simulink model "B5_simulation_paparazzi"  (R2021b)
settings: Solver=VariableStepAuto  StartTime=0.0  StopTime=5.5  FixedStep=0.002  RelTol=1e-3
values from neighbouring files (symbols this model uses):
  coef_sim_1 = tf_des_d.Denominator{1}(2)    [A11_setup_script_pprz.m]    (also in A1_setup_script.m; A6_slow_actuator.m)
  coef_sim_2 = tf_des_d.Numerator{1}(2)    [A11_setup_script_pprz.m]    (also in A1_setup_script.m; A6_slow_actuator.m)
  coeff = 1    [A11_setup_script_pprz.m]    (also in A12_sim_multi_run.m = coeff_list(i))
  doublet_mag = - 0.15    (= -0.15)    [A11_setup_script_pprz.m]    (also in A1_setup_script.m)
  doublet_time = 6    [A11_setup_script_pprz.m]    (also in A1_setup_script.m)
  f_8 = 1    [A11_setup_script_pprz.m]    (also in A1_setup_script.m)
  FILT_CUTOFF = 2*pi*5    (= 31.4159265359)    [A11_setup_script_pprz.m]    (also in A1_setup_script.m)
  FILTER = 1    [A11_setup_script_pprz.m]    (also in A1_setup_script.m)
  G1 = inv(I)*G1_r    [A10_simple_plant.m]    (also in A11_setup_script_pprz.m = G1/scale; A1_setup_script.m = [G1;G1_T])
  G2 = G2/scale    [A11_setup_script_pprz.m]    (also in A1_setup_script.m = (1/sampling_time)*inv(I)*(G2_r))
  h_plate = 0.3    [A11_setup_script_pprz.m]    (also in A1_setup_script.m = 0.16)
  I = eye(3,3)    [A10_simple_plant.m]    (also in A11_setup_script_pprz.m; A1_setup_script.m; A2_B_matrix_generation_symbolic.m = [Ixx 0 0; A3_B_matrix_generation_symbolic_cascaded.m = [Ixx 0 0)
  Iyy = 0.0008    [A11_setup_script_pprz.m]    (also in A1_setup_script.m = 0.0015)
  K = 7    [A11_setup_script_pprz.m]    (also in A1_setup_script.m = 10)
  K_act = 50    [A10_simple_plant.m]    (also in A11_setup_script_pprz.m = 20; A1_setup_script.m = 20)
  K_d = 15    [A11_setup_script_pprz.m]    (also in A1_setup_script.m = 25)
  K_dd = K_act    (= 20)    [A11_setup_script_pprz.m]    (also in A1_setup_script.m)
  K_ec = 50    [A11_setup_script_pprz.m]    (also in A1_setup_script.m = 251)
  K_ec_d = 13    [A11_setup_script_pprz.m]    (also in A1_setup_script.m = 25)
  K_ec_d_u = 1.5    [A11_setup_script_pprz.m]    (also in A1_setup_script.m = 5)
  K_ec_d_v = 1.5    [A11_setup_script_pprz.m]    (also in A1_setup_script.m = 5)
  K_ec_dd = 9    [A11_setup_script_pprz.m]    (also in A1_setup_script.m = 45)
  K_ec_i = 0    [A11_setup_script_pprz.m]    (also in A1_setup_script.m = 380)
  K_ec_u = 1.5    [A11_setup_script_pprz.m]    (also in A1_setup_script.m = 5)
  K_ec_v = 1.5    [A11_setup_script_pprz.m]    (also in A1_setup_script.m = 5)
  K_t = 0.0005    [A10_simple_plant.m]    (also in A11_setup_script_pprz.m = 6.557e-08; A1_setup_script.m = 6.557e-08)
  K_u = 1.0    (= 1)    [A11_setup_script_pprz.m]    (also in A1_setup_script.m = 1.5)
  K_u_d = 2.5    [A11_setup_script_pprz.m]    (also in A1_setup_script.m = 7)
  K_v = 1.0    (= 1)    [A11_setup_script_pprz.m]    (also in A1_setup_script.m = 1.5)
  K_v_d = 2.5    [A11_setup_script_pprz.m]    (also in A1_setup_script.m = 7)
  K_w = 1.0    (= 1)    [A11_setup_script_pprz.m]    (also in A1_setup_script.m = 4.5)
  K_w_d = 2.5    [A11_setup_script_pprz.m]    (also in A1_setup_script.m = 7)
  l_plate = 0.1    [A11_setup_script_pprz.m]    (also in A1_setup_script.m = 0.11)
  m = 0.4    [A10_simple_plant.m]    (also in A11_setup_script_pprz.m; A1_setup_script.m)
  NOISE = 0    [A11_setup_script_pprz.m]    (also in A1_setup_script.m)
  NOISE_ACC = 0.00005    (= 5e-05)    [A11_setup_script_pprz.m]    (also in A1_setup_script.m)
  NOISE_GYRO = 0.00005    (= 5e-05)    [A11_setup_script_pprz.m]    (also in A1_setup_script.m)
  NOISE_RPM = 200    [A11_setup_script_pprz.m]    (also in A1_setup_script.m)
  omega_des = 20.00    (= 20)    [A11_setup_script_pprz.m]    (also in A1_setup_script.m; A6_slow_actuator.m = 49)
  sampling_time = 1/frequency    (= 0.002)    [A11_setup_script_pprz.m]    (also in A12_sim_multi_run.m; A1_setup_script.m; A6_slow_actuator.m)
  scale_8 = 1.6    [A11_setup_script_pprz.m]    (also in A1_setup_script.m)
  start_8 = 2    [A11_setup_script_pprz.m]    (also in A1_setup_script.m)
  start_time = 2    [A11_setup_script_pprz.m]    (also in A1_setup_script.m = 1)
  t_8 = 10    [A11_setup_script_pprz.m]    (also in A1_setup_script.m)
  w_plate = 0.3    [A11_setup_script_pprz.m]    (also in A1_setup_script.m = 0.36)
undefined symbols (not defined in the file or in its folder): DiscIntNeverNeededParam
libraries: simulink x11, cstblocks x9, dspinverses x8, dspmathops x4, dspstat3 x4, aerolibutil x3, sharedutil x2, aerolibanim x1
(part 3 of 5)

== system B5_simulation_paparazzi/Model Block Complementary Filters/Simple INDI/INTERNAL REFERENCE MODEL ATTITUDE ==
  phi_cmd : Inport
  theta_cmd : Inport  Port=2
  psi_cmd : Inport  Port=3
  Discrete-Time Integrator{,1..8} (9 alike) : DiscreteIntegrator  SampleTime=sampling_time  ICPrevOutput=DiscIntNeverNeededParam  ICPrevScaledInput=DiscIntNeverNeededParam
  Gain1 : Gain  Gain=K
  Gain2 : Gain  Gain=K_dd
  Gain3 : Gain  Gain=K
  Gain4 : Gain  Gain=K_d
  Gain5 : Gain  Gain=K_d
  Gain6 : Gain  Gain=K_d
  Gain7 : Gain  Gain=K
  Gain8 : Gain  Gain=K_dd
  Gain9 : Gain  Gain=K_dd
  MATLAB Function1 : MATLAB Function  TreatAsAtomicUnit=on
  Mux : Mux  Inputs=6
  Scope : Scope  NumInputPorts=2
  Sum{1..4,11,16,20..22} (9 alike) : Sum  Inputs=|+-
  To Workspace : ToWorkspace  VariableName=simout  SaveFormat=Timeseries  SampleTime=-1
  body rates to euler rates : Subsystem
  euler rates to body rates : Subsystem
  pd_ref : Outport
  qd_ref : Outport  Port=2
  rd_ref : Outport  Port=3
  p_ref : Outport  Port=4
  q_ref : Outport  Port=5
  r_ref : Outport  Port=6
  phi_ref : Outport  Port=7
  theta_ref : Outport  Port=8
  psi_ref : Outport  Port=9
  tag scope: p_ref=global, phi_ref=global, psi_ref=global, q_ref=global, r_ref=global, theta_ref=global
  wires:
  Discrete-Time Integrator5/1 -> [r_ref], r_ref/1, body rates to euler rates/3(r), Sum22/2  "r_ref"
  [qd_f] -> Mux/4
  MATLAB Function1/1(psie_w) -> Gain3/1  "wrapped_Err"
  Sum22/1 -> Gain6/1
  euler rates to body rates/3(r) -> Sum22/1
  Sum4/1 -> Gain9/1
  Gain1/1 -> euler rates to body rates/2(theta_dot)
  Discrete-Time Integrator7/1 -> Sum3/2, Discrete-Time Integrator4/1, Mux/1, qd_ref/1  "qd_ref"
  Mux/1 -> To Workspace/1
  psi_cmd/1 -> Sum1/1  "psi_cmd"
  Gain9/1 -> Discrete-Time Integrator8/1  "rdd_ref"
  theta_cmd/1 -> Sum11/1  "theta_cmd"
  Gain4/1 -> Sum2/1
  Sum1/1 -> MATLAB Function1/1(pis_e)  "err"
  Discrete-Time Integrator/1 -> [psi_ref], psi_ref/1, Sum1/2  "psi_ref"
  Sum2/1 -> Gain2/1
  Gain3/1 -> euler rates to body rates/3(psi_dot)
  body rates to euler rates/2(theta_dot) -> Scope/2, Discrete-Time Integrator1/1
  Discrete-Time Integrator2/1 -> [phi_ref], phi_ref/1, Sum20/2  "phi_ref"
  Gain6/1 -> Sum4/1
  Sum20/1 -> Gain7/1
  Gain8/1 -> Discrete-Time Integrator7/1  "qdd_ref"
  euler rates to body rates/1(p) -> Sum21/1
  Sum11/1 -> Gain1/1
  Gain2/1 -> Discrete-Time Integrator6/1  "pdd_ref"
  Sum21/1 -> Gain4/1
  Discrete-Time Integrator1/1 -> [theta_ref], Mux/3, theta_ref/1, Sum11/2  "theta_ref"
  Sum3/1 -> Gain8/1
  Gain5/1 -> Sum3/1
  Discrete-Time Integrator6/1 -> Sum2/2, Discrete-Time Integrator3/1, pd_ref/1  "pd_ref"
  euler rates to body rates/2(q) -> Sum16/1
  [theta] -> Mux/6
  Discrete-Time Integrator8/1 -> Sum4/2, Discrete-Time Integrator5/1, rd_ref/1  "rd_ref"
  body rates to euler rates/3(psi_dot) -> Discrete-Time Integrator/1
  phi_cmd/1 -> Sum20/1  "phi_cmd"
  body rates to euler rates/1(phi_dot) -> Discrete-Time Integrator2/1
  [q] -> Mux/5
  Gain7/1 -> euler rates to body rates/1(phi_dot)
  Discrete-Time Integrator3/1 -> [p_ref], p_ref/1, body rates to euler rates/1(p), Sum21/2  "p_ref"
  Discrete-Time Integrator4/1 -> Scope/1, body rates to euler rates/2(q), [q_ref], Mux/2, q_ref/1, Sum16/2  "q_ref"
  Sum16/1 -> Gain5/1

== system B5_simulation_paparazzi/Model Block Complementary Filters/Simple INDI/INTERNAL REFERENCE MODEL VELOCITY ==
  Vx_cmd : Inport
  Vy_cmd : Inport  Port=2
  Vz_cmd : Inport  Port=3
  Discrete-Time Integrator{,1..5} (6 alike) : DiscreteIntegrator  SampleTime=-1  ICPrevOutput=DiscIntNeverNeededParam  ICPrevScaledInput=DiscIntNeverNeededParam
  Gain1 : Gain  Gain=K_w_d
  Gain2 : Gain  Gain=K_v_d
  Gain3 : Gain  Gain=K_w
  Gain4 : Gain  Gain=K_v
  Gain5 : Gain  Gain=K_u
  Gain9 : Gain  Gain=K_u_d
  Sum{1..4,11,20} (6 alike) : Sum  Inputs=|+-
  Ax_ref : Outport
  Ay_ref : Outport  Port=2
  Az_ref : Outport  Port=3
  Vx_ref : Outport  Port=4
  Vy_ref : Outport  Port=5
  Vz_ref : Outport  Port=6
  X_ref : Outport  Port=7
  Y_ref : Outport  Port=8
  Z_ref : Outport  Port=9
  tag scope: Ax_ref=global, Ay_ref=global, Az_ref=global, Vx_ref=global, Vy_ref=global, Vz_ref=global
  wires:
  Discrete-Time Integrator1/1 -> Sum3/2, Discrete-Time Integrator4/1, [Vy_ref], Vz_ref/1
  Gain1/1 -> Discrete-Time Integrator1/1, [Az_ref], Az_ref/1
  Gain9/1 -> Discrete-Time Integrator/1, [Ax_ref], Ax_ref/1
  Vy_cmd/1 -> Sum1/1
  Discrete-Time Integrator/1 -> Sum4/2, Discrete-Time Integrator3/1, [Vx_ref], Vx_ref/1
  Vx_cmd/1 -> Sum20/1
  Vz_cmd/1 -> Sum11/1
  Discrete-Time Integrator2/1 -> Sum2/2, Discrete-Time Integrator5/1, [Vz_ref], Vy_ref/1
  Gain2/1 -> Discrete-Time Integrator2/1, [Ay_ref], Ay_ref/1
  Sum20/1 -> Gain5/1
  Sum11/1 -> Gain3/1
  Sum1/1 -> Gain4/1
  Gain4/1 -> Sum2/1
  Gain3/1 -> Sum3/1
  Gain5/1 -> Sum4/1
  Sum3/1 -> Gain1/1
  Sum2/1 -> Gain2/1
  Sum4/1 -> Gain9/1
  Discrete-Time Integrator3/1 -> X_ref/1, Sum20/2
  Discrete-Time Integrator4/1 -> Sum11/2, Z_ref/1
  Discrete-Time Integrator5/1 -> Sum1/2, Y_ref/1

== system B5_simulation_paparazzi/Model Block Normal Filters/Continuous Actuator Dynamics/Butterworth Lowpass 2nd Order1 ==
  In : Inport
  Constant : Constant  Value=FILTER  SampleTime=sampling_time
  Merge : Merge
  Switch Case : SwitchCase
  Switch Case Action Subsystem : Subsystem  TreatAsAtomicUnit=on
  Switch Case Action Subsystem1 : Subsystem  TreatAsAtomicUnit=on
  Out : Outport
  wires:
  Merge/1 -> Out/1
  Switch Case Action Subsystem/1(Out1) -> Merge/1
  Constant/1 -> Switch Case/1
  Switch Case Action Subsystem1/1(Out1) -> Merge/2
  Switch Case/2 -> Switch Case Action Subsystem1/Action
  In/1 -> Switch Case Action Subsystem/1(In1), Switch Case Action Subsystem1/1(In1)
  Switch Case/1 -> Switch Case Action Subsystem/Action

== system B5_simulation_paparazzi/Model Block Normal Filters/Continuous Actuator Dynamics/Noise RPM ==
  Constant : Constant  Value=NOISE  SampleTime=sampling_time
  Merge : Merge
  Switch Case : SwitchCase
  Switch Case Action Subsystem : Subsystem  TreatAsAtomicUnit=on
  Switch Case Action Subsystem1 : Subsystem  TreatAsAtomicUnit=on
  Out : Outport
  wires:
  Switch Case/2 -> Switch Case Action Subsystem1/Action
  Merge/1 -> Out/1
  Switch Case/1 -> Switch Case Action Subsystem/Action
  Constant/1 -> Switch Case/1
  Switch Case Action Subsystem1/1(Out1) -> Merge/2
  Switch Case Action Subsystem/1(Out1) -> Merge/1

== system B5_simulation_paparazzi/Model Block Normal Filters/Extended INDI/8-shape trajectory ==
  Abs : Abs
  Abs1 : Abs
  Clock : Clock
      settings: Decimation=100
  Constant : Constant  Value=f_8
  Constant1 : Constant  Value=scale_8
  Constant2 : Constant  Value=t_8
  Constant3 : Constant  Value=sampling_time
  Constant4 : Constant  Value=0
  Constant5 : Constant  Value=start_8
  Constant6 : Constant  Value=t_8
  Constant7 : Constant  Value=start_8
  Integrator : Integrator
  MATLAB Function : MATLAB Function  TreatAsAtomicUnit=on
  Scope : Scope
  Scope1 : Scope
  Sum : Sum  Inputs=|+-
  Sum3 : Sum  Inputs=|+-
  Sum7 : Sum  Inputs=|+-
  Sum9 : Sum  Inputs=|++
  Switch : Switch  Criteria=u2 > Threshold  Threshold=t_8
  Switch1 : Switch  Criteria=u2 > Threshold  Threshold=start_8
  Zero-Order Hold : ZeroOrderHold  SampleTime=sampling_time
  x_traj : Outport
  y_traj : Outport  Port=2
  psi_traj : Outport  Port=3
  wires:
  Constant2/1 -> Switch/1
  Switch/1 -> Scope/1, MATLAB Function/1(t)  "t"
  Constant/1 -> MATLAB Function/2(f)
  MATLAB Function/2(y) -> y_traj/1, Sum7/2  "y_traj"
  Zero-Order Hold/1 -> Switch/2, Switch/3
  Constant1/1 -> MATLAB Function/3(scale)
  Constant3/1 -> MATLAB Function/4(sampling_time)
  MATLAB Function/1(x) -> x_traj/1, Sum3/2  "x_traj"
  MATLAB Function/3(psi) -> psi_traj/1  "psi_traj"
  Clock/1 -> Sum/1, Switch1/2
  Constant4/1 -> Switch1/3
  Switch1/1 -> Zero-Order Hold/1
  Constant5/1 -> Sum/2
  Sum/1 -> Switch1/1
  Constant6/1 -> MATLAB Function/5(total_time)
  Sum7/1 -> Abs1/1
  Abs/1 -> Sum9/1
  Abs1/1 -> Sum9/2
  [y] -> Sum7/1
  Sum9/1 -> Integrator/1
  Integrator/1 -> Scope1/1  "pos_err"
  [x] -> Sum3/1
  Sum3/1 -> Abs/1
  Constant7/1 -> MATLAB Function/6(start_time)

== system B5_simulation_paparazzi/Model Block Normal Filters/Extended INDI/Doublet Block ==
  Scope : Scope
  Step : Step  Time=start_time  After=doublet_mag  SampleTime=sampling_time
  Step1 : Step  Time=start_time + doublet_time/2  After=-doublet_mag*2  SampleTime=sampling_time
  Step2 : Step  Time=start_time + doublet_time  After=doublet_mag  SampleTime=sampling_time
  Sum : Sum  Inputs=|++
  Sum1 : Sum  Inputs=|++
  theta_cmd : Outport
  wires:
  Step/1 -> Sum/1
  Step1/1 -> Sum/2
  Sum/1 -> Sum1/1
  Sum1/1 -> theta_cmd/1, Scope/1
  Step2/1 -> Sum1/2

== system B5_simulation_paparazzi/Model Block Normal Filters/Extended INDI/ERROR CONTROLLER ATTITUDE ==
  pd_ref : Inport
  qd_ref : Inport  Port=2
  rd_ref : Inport  Port=3
  p_ref : Inport  Port=4
  q_ref : Inport  Port=5
  r_ref : Inport  Port=6
  phi_ref : Inport  Port=7
  theta_ref : Inport  Port=8
  psi_ref : Inport  Port=9
  Abs : Abs
  Add : Sum  Inputs=++++
  Add1 : Sum  Inputs=++++
  Add2 : Sum  Inputs=++++
  Cumulative Sum : dspmathops/Cumulative Sum  dim=Channels (running sum)  InputProcessing=Columns as channels (frame based)  reset_popup=None  roundingMode=Floor  overflowMode=off  outputDataTypeStr=Inherit: Same as accumulator  outputMin=[]  outputMax=[]  outputLastDataTypeStr=Inherit: Same as accumulator
  Display : Display
  Display1 : Display
  Gain : Gain  Gain=K_ec_dd + K_act
  Gain1 : Gain  Gain=K_ec_d *(1 + K_act)
  Gain2 : Gain  Gain=K_ec*(1 + K_act)
  Gain3 : Gain  Gain=K_ec_dd + K_act
  Gain4 : Gain  Gain=K_ec_d *(1 + K_act)
  Gain5 : Gain  Gain=K_ec *(1 + K_act)
  Gain6 : Gain  Gain=K_ec_dd + K_act
  Gain7 : Gain  Gain=K_ec_d *(1 + K_act)
  Gain8 : Gain  Gain=K_ec *(1 + K_act)
  MATLAB Function1 : MATLAB Function  TreatAsAtomicUnit=on
  Mean : dspstat3/Mean  run=off  InputProcessing=Columns as channels (frame based)  reset_popup=None  directionMode=Each column  dimension=1  roiEnable=off  roiType=Rectangles  roiPortion=Entire ROI  roiOutput=Individual statistics for each ROI  roiFlag=off  roundingMode=Floor  overflowMode=off  outputDataTypeStr=Inherit: Same as accumulator  outputMin=[]  outputMax=[]  outputLastDataTypeStr=Inherit: Same as accumulator
  Scope : Scope  NumInputPorts=4
  Sum{,1..8} (9 alike) : Sum  Inputs=|+-
  pdd_ec : Outport
  qdd_ec : Outport  Port=2
  rdd_ec : Outport  Port=3
  wires:
  pd_ref/1 -> Sum/1
  p_ref/1 -> Sum1/1
  Add/1 -> pdd_ec/1
  [p] -> Sum1/2
  [phi] -> Sum2/2
  phi_ref/1 -> Sum2/1
  [pd_f] -> Sum/2
  Sum/1 -> Gain/1  "pd_err"
  Gain/1 -> Add/1
  Sum1/1 -> Gain1/1  "p_err"
  Sum2/1 -> Gain2/1  "phi_err"
  Gain1/1 -> Add/2
  Gain2/1 -> Add/3
  Sum4/1 -> Gain4/1  "q_err"
  [qd_f] -> Sum3/2
  Gain4/1 -> Add1/2
  Gain5/1 -> Add1/3
  theta_ref/1 -> Sum5/1
  [theta] -> Sum5/2
  [q] -> Sum4/2
  Gain3/1 -> Add1/1
  q_ref/1 -> Sum4/1
  Add1/1 -> qdd_ec/1
  qd_ref/1 -> Sum3/1
  Sum7/1 -> Gain7/1  "r_err"
  Sum8/1 -> MATLAB Function1/1(pis_e)
  Sum6/1 -> Gain6/1  "rd_err"
  [rd_f] -> Sum6/2
  Gain7/1 -> Scope/2, Add2/2  "2"
  Gain8/1 -> Scope/3, Add2/3  "3"
  psi_ref/1 -> Sum8/1
  [psi] -> Sum8/2
  [r] -> Sum7/2
  Gain6/1 -> Add2/1, Scope/1  "1"
  r_ref/1 -> Sum7/1
  Add2/1 -> rdd_ec/1
  rd_ref/1 -> Sum6/1
  Sum3/1 -> Gain3/1  "qd_err"
  Sum5/1 -> Abs/1, Gain5/1  "theta_err"
  MATLAB Function1/1(psie_w) -> Gain8/1  "psi_err"
  Abs/1 -> Mean/1, Cumulative Sum/1  "theta_err_abs"
  Cumulative Sum/1 -> Display/1
  Mean/1 -> Display1/1

== system B5_simulation_paparazzi/Model Block Normal Filters/Extended INDI/ERROR CONTROLLER VELOCITY ==
  Vx_ref : Inport
  Vy_ref : Inport  Port=2
  Vz_ref : Inport  Port=3
  X_ref : Inport  Port=4
  Y_ref : Inport  Port=5
  Z_ref : Inport  Port=6
  Gain : Gain  Gain=K_ec_u
  Gain1 : Gain  Gain=K_ec_d_u
  Gain2 : Gain  Gain=K_ec_v
  Gain3 : Gain  Gain=K_ec_d_v
  Gain4 : Gain  Gain=K_ec_v
  Gain5 : Gain  Gain=K_ec_d_v
  Sum{,3,5..8} (6 alike) : Sum  Inputs=|+-
  Sum1 : Sum  Inputs=|++
  Sum2 : Sum  Inputs=|++
  Sum4 : Sum  Inputs=|++
  Ax_ec : Outport
  Ay_ec : Outport  Port=2
  Az_ec : Outport  Port=3
  wires:
  [Vz] -> Sum6/2
  Sum1/1 -> Ax_ec/1
  Sum2/1 -> Ay_ec/1
  Vy_ref/1 -> Sum3/1
  Vx_ref/1 -> Sum/1
  [Vy] -> Sum3/2
  Vz_ref/1 -> Sum6/1
  Sum/1 -> Gain1/1  "Vx_error"
  Sum4/1 -> Az_ec/1
  [Vx] -> Sum/2
  [x] -> Sum5/2
  X_ref/1 -> Sum5/1
  Sum5/1 -> Gain/1
  Gain1/1 -> Sum1/1
  Gain/1 -> Sum1/2
  Gain3/1 -> Sum2/1
  Sum3/1 -> Gain3/1  "Vy_error"
  Gain5/1 -> Sum4/1
  Sum6/1 -> Gain5/1  "Vz_error"
  Y_ref/1 -> Sum7/1
  [y] -> Sum7/2
  Sum7/1 -> Gain2/1
  Z_ref/1 -> Sum8/1
  [z] -> Sum8/2
  Sum8/1 -> Gain4/1
  Gain4/1 -> Sum4/2
  Gain2/1 -> Sum2/2

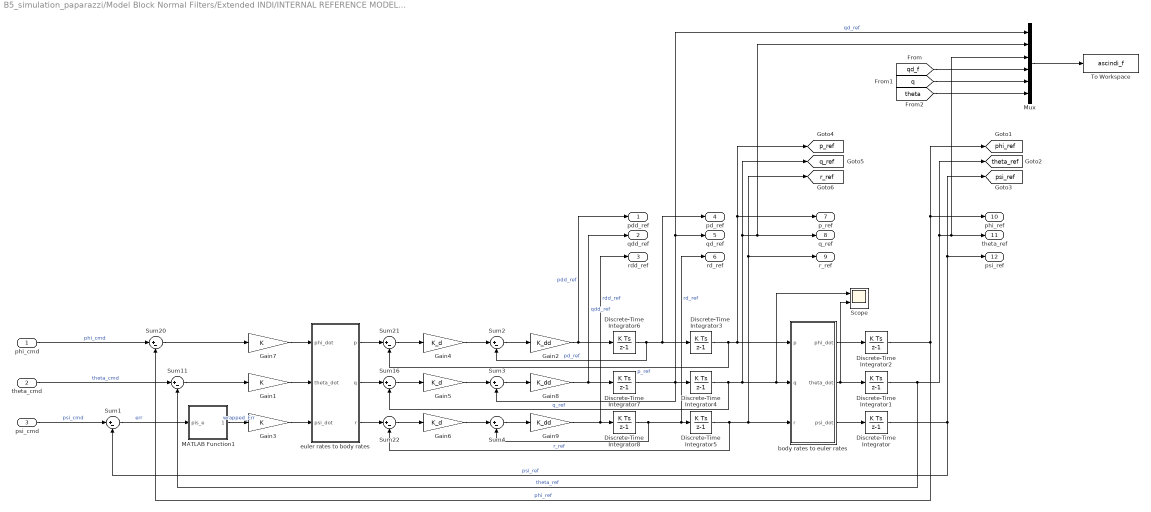
== system B5_simulation_paparazzi/Model Block Normal Filters/Extended INDI/INTERNAL REFERENCE MODEL ATTITUDE ==
  phi_cmd : Inport
  theta_cmd : Inport  Port=2
  psi_cmd : Inport  Port=3
  Discrete-Time Integrator{,1..8} (9 alike) : DiscreteIntegrator  SampleTime=sampling_time  ICPrevOutput=DiscIntNeverNeededParam  ICPrevScaledInput=DiscIntNeverNeededParam
  Gain1 : Gain  Gain=K
  Gain2 : Gain  Gain=K_dd
  Gain3 : Gain  Gain=K
  Gain4 : Gain  Gain=K_d
  Gain5 : Gain  Gain=K_d
  Gain6 : Gain  Gain=K_d
  Gain7 : Gain  Gain=K
  Gain8 : Gain  Gain=K_dd
  Gain9 : Gain  Gain=K_dd
  MATLAB Function1 : MATLAB Function  TreatAsAtomicUnit=on
  Mux : Mux  Inputs=6
  Scope : Scope  NumInputPorts=2
  Sum{1..4,11,16,20..22} (9 alike) : Sum  Inputs=|+-
  To Workspace : ToWorkspace  VariableName=ascindi_f  SaveFormat=Timeseries  SampleTime=-1
  body rates to euler rates : Subsystem
  euler rates to body rates : Subsystem
  pdd_ref : Outport
  qdd_ref : Outport  Port=2
  rdd_ref : Outport  Port=3
  pd_ref : Outport  Port=4
  qd_ref : Outport  Port=5
  rd_ref : Outport  Port=6
  p_ref : Outport  Port=7
  q_ref : Outport  Port=8
  r_ref : Outport  Port=9
  phi_ref : Outport  Port=10
  theta_ref : Outport  Port=11
  psi_ref : Outport  Port=12
  tag scope: p_ref=global, phi_ref=global, psi_ref=global, q_ref=global, r_ref=global, theta_ref=global
  wires:
  Discrete-Time Integrator1/1 -> [theta_ref], Mux/3, theta_ref/1, Sum11/2  "theta_ref"
  Discrete-Time Integrator8/1 -> Sum4/2, Discrete-Time Integrator5/1, rd_ref/1  "rd_ref"
  Discrete-Time Integrator3/1 -> [p_ref], p_ref/1, body rates to euler rates/1(p), Sum21/2  "p_ref"
  Discrete-Time Integrator5/1 -> [r_ref], r_ref/1, body rates to euler rates/3(r), Sum22/2  "r_ref"
  Discrete-Time Integrator4/1 -> Scope/1, body rates to euler rates/2(q), [q_ref], Mux/2, q_ref/1, Sum16/2  "q_ref"
  Discrete-Time Integrator7/1 -> Sum3/2, Discrete-Time Integrator4/1, Mux/1, qd_ref/1  "qd_ref"
  Sum21/1 -> Gain4/1
  Sum11/1 -> Gain1/1
  Sum22/1 -> Gain6/1
  Sum16/1 -> Gain5/1
  Discrete-Time Integrator2/1 -> [phi_ref], phi_ref/1, Sum20/2  "phi_ref"
  Sum20/1 -> Gain7/1
  Discrete-Time Integrator6/1 -> Sum2/2, Discrete-Time Integrator3/1, pd_ref/1  "pd_ref"
  phi_cmd/1 -> Sum20/1  "phi_cmd"
  theta_cmd/1 -> Sum11/1  "theta_cmd"
  psi_cmd/1 -> Sum1/1  "psi_cmd"
  Discrete-Time Integrator/1 -> [psi_ref], psi_ref/1, Sum1/2  "psi_ref"
  Sum1/1 -> MATLAB Function1/1(pis_e)  "err"
  Gain4/1 -> Sum2/1
  Gain5/1 -> Sum3/1
  Gain6/1 -> Sum4/1
  Sum2/1 -> Gain2/1
  Sum3/1 -> Gain8/1
  Sum4/1 -> Gain9/1
  Gain2/1 -> Discrete-Time Integrator6/1, pdd_ref/1  "pdd_ref"
  Gain8/1 -> Discrete-Time Integrator7/1, qdd_ref/1  "qdd_ref"
  Gain9/1 -> Discrete-Time Integrator8/1, rdd_ref/1  "rdd_ref"
  Gain7/1 -> euler rates to body rates/1(phi_dot)
  euler rates to body rates/1(p) -> Sum21/1
  Gain1/1 -> euler rates to body rates/2(theta_dot)
  euler rates to body rates/2(q) -> Sum16/1
  Gain3/1 -> euler rates to body rates/3(psi_dot)
  euler rates to body rates/3(r) -> Sum22/1
  body rates to euler rates/3(psi_dot) -> Discrete-Time Integrator/1
  body rates to euler rates/2(theta_dot) -> Scope/2, Discrete-Time Integrator1/1
  body rates to euler rates/1(phi_dot) -> Discrete-Time Integrator2/1
  MATLAB Function1/1(psie_w) -> Gain3/1  "wrapped_Err"
  Mux/1 -> To Workspace/1
  [qd_f] -> Mux/4
  [theta] -> Mux/6
  [q] -> Mux/5

== system B5_simulation_paparazzi/Model Block Normal Filters/Extended INDI/INTERNAL REFERENCE MODEL VELOCITY ==
  Vx_cmd : Inport
  Vy_cmd : Inport  Port=2
  Vz_cmd : Inport  Port=3
  Discrete-Time Integrator{,1..5} (6 alike) : DiscreteIntegrator  SampleTime=-1  ICPrevOutput=DiscIntNeverNeededParam  ICPrevScaledInput=DiscIntNeverNeededParam
  Gain1 : Gain  Gain=K_w_d
  Gain2 : Gain  Gain=K_v_d
  Gain3 : Gain  Gain=K_w
  Gain4 : Gain  Gain=K_v
  Gain5 : Gain  Gain=K_u
  Gain9 : Gain  Gain=K_u_d
  Sum{1..4,11,20} (6 alike) : Sum  Inputs=|+-
  Ax_ref : Outport
  Ay_ref : Outport  Port=2
  Az_ref : Outport  Port=3
  Vx_ref : Outport  Port=4
  Vy_ref : Outport  Port=5
  Vz_ref : Outport  Port=6
  X_ref : Outport  Port=7
  Y_ref : Outport  Port=8
  Z_ref : Outport  Port=9
  tag scope: Ax_ref=global, Ay_ref=global, Az_ref=global, Vx_ref=global, Vy_ref=global, Vz_ref=global
  wires:
  Discrete-Time Integrator1/1 -> Sum3/2, Discrete-Time Integrator4/1, [Vy_ref], Vz_ref/1
  Gain1/1 -> Discrete-Time Integrator1/1, [Az_ref], Az_ref/1
  Gain9/1 -> Discrete-Time Integrator/1, [Ax_ref], Ax_ref/1
  Vy_cmd/1 -> Sum1/1
  Discrete-Time Integrator/1 -> Sum4/2, Discrete-Time Integrator3/1, [Vx_ref], Vx_ref/1
  Vx_cmd/1 -> Sum20/1
  Vz_cmd/1 -> Sum11/1
  Discrete-Time Integrator2/1 -> Sum2/2, Discrete-Time Integrator5/1, [Vz_ref], Vy_ref/1
  Gain2/1 -> Discrete-Time Integrator2/1, [Ay_ref], Ay_ref/1
  Sum20/1 -> Gain5/1
  Sum11/1 -> Gain3/1
  Sum1/1 -> Gain4/1
  Gain4/1 -> Sum2/1
  Gain3/1 -> Sum3/1
  Gain5/1 -> Sum4/1
  Sum3/1 -> Gain1/1
  Sum2/1 -> Gain2/1
  Sum4/1 -> Gain9/1
  Discrete-Time Integrator3/1 -> X_ref/1, Sum20/2
  Discrete-Time Integrator4/1 -> Sum11/2, Z_ref/1
  Discrete-Time Integrator5/1 -> Sum1/2, Y_ref/1

== system B5_simulation_paparazzi/Model Block Normal Filters/Extended INDI/Subsystem ==
  Constant : Constant  Value=w_plate
  Constant1 : Constant  Value=Iyy
  Constant2 : Constant  Value=l_plate
  Constant3 : Constant  Value=h_plate
  MATLAB Function : MATLAB Function  TreatAsAtomicUnit=on
  Terminator : Terminator
  Terminator1 : Terminator
  body rates to euler rates : Subsystem
  qdd_comp : Outport
  wires:
  MATLAB Function/1(qdd_comp) -> qdd_comp/1  "qdd_comp"
  [theta] -> MATLAB Function/1(theta)
  [Vx] -> MATLAB Function/3(Vx)
  [Ax] -> MATLAB Function/6(Ax)
  Constant/1 -> MATLAB Function/10(w_plate)
  Constant1/1 -> MATLAB Function/13(Iyy)
  Constant2/1 -> MATLAB Function/12(l_plate)
  Constant3/1 -> MATLAB Function/11(h_plate)
  [p] -> body rates to euler rates/1(p)
  [q] -> body rates to euler rates/2(q)
  [r] -> body rates to euler rates/3(r)
  body rates to euler rates/2(theta_dot) -> MATLAB Function/2(dtheta)
  body rates to euler rates/1(phi_dot) -> Terminator/1
  [Vy] -> MATLAB Function/4(Vy)
  [Ay] -> MATLAB Function/7(Ay)
  body rates to euler rates/3(psi_dot) -> Terminator1/1
  [u_cont] -> MATLAB Function/9(u)
  [Vz] -> MATLAB Function/5(Vz)
  [Az] -> MATLAB Function/8(Az)

== system B5_simulation_paparazzi/Model Block Normal Filters/Force and Moment Calculation/Drag Plate Aerodynamics ==
  Constant : Constant  Value=0  SampleTime=sampling_time
  Constant1 : Constant  Value=w_plate
  Constant4 : Constant  Value=h_plate
  Constant6 : Constant  Value=l_plate
  Mux : Mux  Inputs=3
  Scope1 : Scope  NumInputPorts=3
  Scope2 : Scope  NumInputPorts=2
  Scope3 : Scope  NumInputPorts=3
  Scope4 : Scope
  Scope5 : Scope  NumInputPorts=3
  drag plate My1 : MATLAB Function  TreatAsAtomicUnit=on
  aero_moment : Outport
  wires:
  Constant4/1 -> drag plate My1/2(h_plate)
  Constant6/1 -> drag plate My1/3(l_plate)
  [theta_cont] -> drag plate My1/4("theta ")
  Constant1/1 -> drag plate My1/1(w_plate)
  [Vy_cont] -> drag plate My1/6("Vy ")
  [Vx_cont] -> drag plate My1/5("Vx ")
  drag plate My1/6(gamma) -> Scope1/1  "gamma"
  [Vz_cont] -> drag plate My1/7("Vz ")
  drag plate My1/7(theta) -> Scope1/2  "theta_deg"
  drag plate My1/8(alpha) -> Scope1/3  "alpha"
  drag plate My1/1(Cd) -> Scope2/1  "Cd"
  drag plate My1/2(Cl) -> Scope2/2  "Cl"
  drag plate My1/9(D_plate) -> Scope3/1  "D_plate"
  drag plate My1/10(L_plate) -> Scope3/2  "L_plate"
  [u_cont] -> drag plate My1/8(u)
  drag plate My1/12(My_dp) -> Mux/2, Scope4/1  "My_dp"
  drag plate My1/3(Vx) -> Scope5/1  "Vx"
  drag plate My1/4(Vy) -> Scope5/2  "Vy"
  drag plate My1/5(Vz) -> Scope5/3  "Vz"
  Constant/1 -> Mux/1, Mux/3
  Mux/1 -> aero_moment/1
  drag plate My1/11(R_plate) -> Scope3/3  "R_plate"

== system B5_simulation_paparazzi/Model Block Normal Filters/Plant and State Estimation/Butterworth Lowpass 2nd Order1 ==
  In : Inport
  Constant : Constant  Value=FILTER  SampleTime=sampling_time
  Merge : Merge
  Switch Case : SwitchCase
  Switch Case Action Subsystem : Subsystem  TreatAsAtomicUnit=on
  Switch Case Action Subsystem1 : Subsystem  TreatAsAtomicUnit=on
  Out : Outport
  wires:
  Merge/1 -> Out/1
  Switch Case Action Subsystem/1(Out1) -> Merge/1
  Constant/1 -> Switch Case/1
  Switch Case Action Subsystem1/1(Out1) -> Merge/2
  Switch Case/2 -> Switch Case Action Subsystem1/Action
  In/1 -> Switch Case Action Subsystem/1(In1), Switch Case Action Subsystem1/1(In1)
  Switch Case/1 -> Switch Case Action Subsystem/Action

== system B5_simulation_paparazzi/Model Block Normal Filters/Plant and State Estimation/Butterworth Lowpass 2nd Order2 ==
  In : Inport
  Constant : Constant  Value=FILTER  SampleTime=sampling_time
  Merge : Merge
  Switch Case : SwitchCase
  Switch Case Action Subsystem : Subsystem  TreatAsAtomicUnit=on
  Switch Case Action Subsystem1 : Subsystem  TreatAsAtomicUnit=on
  Out : Outport
  wires:
  Merge/1 -> Out/1
  Switch Case Action Subsystem/1(Out1) -> Merge/1
  Constant/1 -> Switch Case/1
  Switch Case Action Subsystem1/1(Out1) -> Merge/2
  Switch Case/2 -> Switch Case Action Subsystem1/Action
  In/1 -> Switch Case Action Subsystem/1(In1), Switch Case Action Subsystem1/1(In1)
  Switch Case/1 -> Switch Case Action Subsystem/Action

== system B5_simulation_paparazzi/Model Block Normal Filters/Plant and State Estimation/Butterworth Lowpass 2nd Order3 ==
  In : Inport
  Constant : Constant  Value=FILTER  SampleTime=sampling_time
  Merge : Merge
  Switch Case : SwitchCase
  Switch Case Action Subsystem : Subsystem  TreatAsAtomicUnit=on
  Switch Case Action Subsystem1 : Subsystem  TreatAsAtomicUnit=on
  Out : Outport
  wires:
  Merge/1 -> Out/1
  Switch Case Action Subsystem/1(Out1) -> Merge/1
  Constant/1 -> Switch Case/1
  Switch Case Action Subsystem1/1(Out1) -> Merge/2
  Switch Case/2 -> Switch Case Action Subsystem1/Action
  In/1 -> Switch Case Action Subsystem/1(In1), Switch Case Action Subsystem1/1(In1)
  Switch Case/1 -> Switch Case Action Subsystem/Action

== system B5_simulation_paparazzi/Model Block Normal Filters/Plant and State Estimation/Butterworth Lowpass 2nd Order4 ==
  In : Inport
  Constant : Constant  Value=FILTER  SampleTime=sampling_time
  Merge : Merge
  Switch Case : SwitchCase
  Switch Case Action Subsystem : Subsystem  TreatAsAtomicUnit=on
  Switch Case Action Subsystem1 : Subsystem  TreatAsAtomicUnit=on
  Out : Outport
  wires:
  Merge/1 -> Out/1
  Switch Case Action Subsystem/1(Out1) -> Merge/1
  Constant/1 -> Switch Case/1
  Switch Case Action Subsystem1/1(Out1) -> Merge/2
  Switch Case/2 -> Switch Case Action Subsystem1/Action
  In/1 -> Switch Case Action Subsystem/1(In1), Switch Case Action Subsystem1/1(In1)
  Switch Case/1 -> Switch Case Action Subsystem/Action

== system B5_simulation_paparazzi/Model Block Normal Filters/Plant and State Estimation/Noise Acc ==
  Constant : Constant  Value=NOISE  SampleTime=sampling_time
  Merge : Merge
  Switch Case : SwitchCase
  Switch Case Action Subsystem : Subsystem  TreatAsAtomicUnit=on
  Switch Case Action Subsystem1 : Subsystem  TreatAsAtomicUnit=on
  Out : Outport
  wires:
  Switch Case/2 -> Switch Case Action Subsystem1/Action
  Merge/1 -> Out/1
  Switch Case/1 -> Switch Case Action Subsystem/Action
  Constant/1 -> Switch Case/1
  Switch Case Action Subsystem1/1(Out1) -> Merge/2
  Switch Case Action Subsystem/1(Out1) -> Merge/1

== system B5_simulation_paparazzi/Model Block Normal Filters/Plant and State Estimation/Noise Gyro ==
  Constant : Constant  Value=NOISE  SampleTime=sampling_time
  Merge : Merge
  Switch Case : SwitchCase
  Switch Case Action Subsystem : Subsystem  TreatAsAtomicUnit=on
  Switch Case Action Subsystem1 : Subsystem  TreatAsAtomicUnit=on
  Out : Outport
  wires:
  Switch Case/2 -> Switch Case Action Subsystem1/Action
  Merge/1 -> Out/1
  Switch Case/1 -> Switch Case Action Subsystem/Action
  Constant/1 -> Switch Case/1
  Switch Case Action Subsystem1/1(Out1) -> Merge/2
  Switch Case Action Subsystem/1(Out1) -> Merge/1

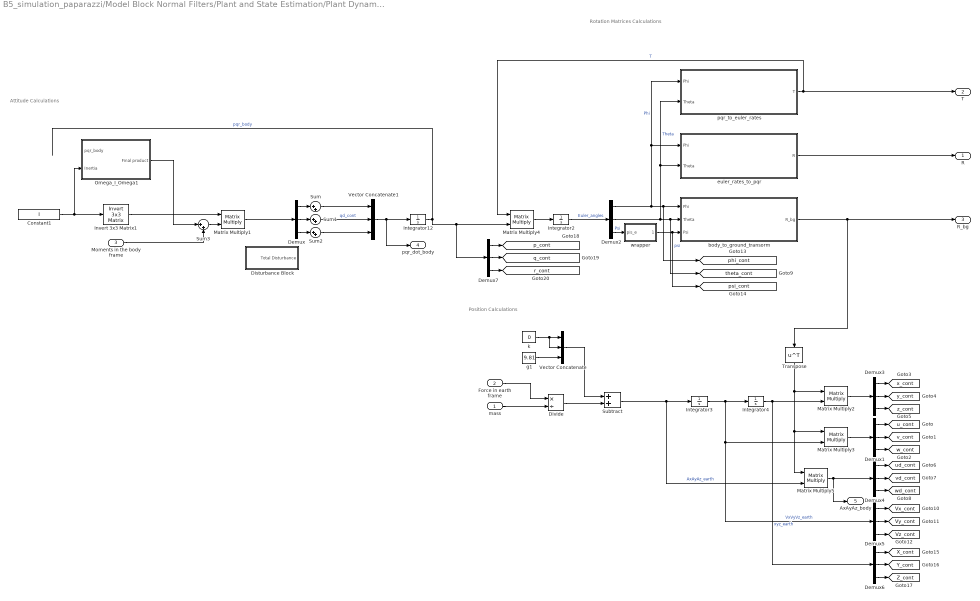
== system B5_simulation_paparazzi/Model Block Normal Filters/Plant and State Estimation/Plant Dynamics Continuous ==
  note: Attitude Calculations
  note: Rotation Matrices Calculations
  note: Position Calculations
  mass : Inport
  Force in earth frame : Inport  Port=2
  Moments in the body frame : Inport  Port=3
  Constant1 : Constant  Value=I  SampleTime=sampling_time
  Demux{,1..7} (8 alike) : Demux  Outputs=3
  Disturbance Block : Subsystem
  Divide : Product  Inputs=*/
  Integrator{2..4,12} (4 alike) : Integrator
  Invert 3x3 Matrix1 : aerolibutil/Invert  3x3 Matrix
  Matrix Multiply{1..5} (5 alike) : Product  Multiplication=Matrix(*)
  Omega_I_Omega1 : Subsystem
  Subtract : Sum
  Sum{,1..3} (4 alike) : Sum  Inputs=|++
  Transpose : Math  Operator=transpose  SaturateOnIntegerOverflow=on
  Vector Concatenate : Concatenate  NumInputs=3
  Vector Concatenate1 : Concatenate  NumInputs=3
  body_to_ground_transorm : MATLAB Function  Description=|  TreatAsAtomicUnit=on
      | This function computes the rotational matrix to pass from the body frame to the world frame. 
      | Takes as inpout the euler angles.
  euler_rates_to_pqr : MATLAB Function  TreatAsAtomicUnit=on
  g1 : Constant  Value=9.81  VectorParams1D=off
  k : Constant  Value=0  VectorParams1D=off
  pqr_to_euler_rates : MATLAB Function  TreatAsAtomicUnit=on
  wrapper : MATLAB Function  TreatAsAtomicUnit=on
  R : Outport
  T : Outport  Port=2
  R_bg : Outport  Port=3
  pqr_dot_body : Outport  Port=4
  AxAyAz_body : Outport  Port=5
  tag scope: Vx_cont=global, Vy_cont=global, Vz_cont=global, X_cont=global, Y_cont=global, Z_cont=global, p_cont=global, phi_cont=global, psi_cont=global, q_cont=global, r_cont=global, theta_cont=global, u_cont=global, ud_cont=global, v_cont=global, vd_cont=global, w_cont=global, wd_cont=global, x_cont=global, y_cont=global, z_cont=global
  wires:
  Demux/1 -> Sum/1
  Sum2/1 -> Vector Concatenate1/3
  Integrator2/1 -> Demux2/1  "Euler_angles"
  Integrator12/1 -> Demux7/1, Matrix Multiply4/2  "pqr_body"
  Divide/1 -> Subtract/2
  Matrix Multiply5/1 -> AxAyAz_body/1, Demux4/1
  mass/1 -> Divide/2
  Integrator4/1 -> Demux6/1, Matrix Multiply2/2  "xyz_earth"
  Demux2/1 -> pqr_to_euler_rates/1(Phi), euler_rates_to_pqr/1(Phi), [phi_cont], body_to_ground_transorm/1(Phi)  "Phi"
  Vector Concatenate1/1 -> Integrator12/1, pqr_dot_body/1
  Demux/2 -> Sum1/1
  Matrix Multiply3/1 -> Demux1/1
  Demux/3 -> Sum2/1
  Transpose/1 -> Matrix Multiply2/1, Matrix Multiply3/1, Matrix Multiply5/1
  k/1 -> Vector Concatenate/2, Vector Concatenate/1
  Vector Concatenate/1 -> Subtract/1
  pqr_to_euler_rates/1(T) -> T/1, Matrix Multiply4/1  "T"
  Subtract/1 -> Integrator3/1, Matrix Multiply5/2  "AxAyAz_earth"
  Integrator3/1 -> Matrix Multiply3/2, Demux5/1, Integrator4/1  "VxVyVz_earth"
  Matrix Multiply2/1 -> Demux3/1
  Force in earth frame/1 -> Divide/1
  Demux2/3 -> wrapper/1(pis_e)  "Psi"
  Sum/1 -> Vector Concatenate1/1
  Sum1/1 -> Vector Concatenate1/2  "qd_cont"
  body_to_ground_transorm/1(R_bg) -> Transpose/1, R_bg/1
  g1/1 -> Vector Concatenate/3
  Constant1/1 -> Invert 3x3 Matrix1/1, Omega_I_Omega1/2(Inertia)
  Moments in the body frame/1 -> Sum3/2
  euler_rates_to_pqr/1(R) -> R/1
  Invert 3x3 Matrix1/1 -> Matrix Multiply1/1
  Matrix Multiply1/1 -> Demux/1
  Demux1/1 -> [u_cont]
  Demux1/2 -> [v_cont]
  Demux1/3 -> [w_cont]
  Demux3/1 -> [x_cont]
  Demux3/2 -> [y_cont]
  Demux3/3 -> [z_cont]
  Demux4/1 -> [ud_cont]
  Demux4/2 -> [vd_cont]
  Demux4/3 -> [wd_cont]
  Sum3/1 -> Matrix Multiply1/2
  Omega_I_Omega1/1(Final product) -> Sum3/1
  Matrix Multiply4/1 -> Integrator2/1
  Demux2/2 -> [theta_cont], body_to_ground_transorm/2(Theta), pqr_to_euler_rates/2(Theta), euler_rates_to_pqr/2(Theta)  "Theta"
  wrapper/1(psie_w) -> [psi_cont], body_to_ground_transorm/3(Psi)  "psi"
  Demux5/1 -> [Vx_cont]
  Demux5/2 -> [Vy_cont]
  Demux5/3 -> [Vz_cont]
  Demux6/1 -> [X_cont]
  Demux6/2 -> [Y_cont]
  Demux6/3 -> [Z_cont]
  Demux7/1 -> [p_cont]
  Demux7/2 -> [q_cont]
  Demux7/3 -> [r_cont]

== system B5_simulation_paparazzi/Model Block Normal Filters/Simple INDI/8-shape trajectory ==
  Abs : Abs
  Abs1 : Abs
  Clock : Clock
      settings: Decimation=100
  Constant : Constant  Value=f_8
  Constant1 : Constant  Value=scale_8
  Constant2 : Constant  Value=t_8
  Constant3 : Constant  Value=sampling_time
  Constant4 : Constant  Value=0
  Constant5 : Constant  Value=start_8
  Constant6 : Constant  Value=t_8
  Constant7 : Constant  Value=start_8
  Integrator : Integrator
  MATLAB Function : MATLAB Function  TreatAsAtomicUnit=on
  Scope : Scope
  Scope1 : Scope
  Sum : Sum  Inputs=|+-
  Sum3 : Sum  Inputs=|+-
  Sum7 : Sum  Inputs=|+-
  Sum9 : Sum  Inputs=|++
  Switch : Switch  Criteria=u2 > Threshold  Threshold=t_8
  Switch1 : Switch  Criteria=u2 > Threshold  Threshold=start_8
  Zero-Order Hold : ZeroOrderHold  SampleTime=sampling_time
  x_traj : Outport
  y_traj : Outport  Port=2
  psi_traj : Outport  Port=3
  wires:
  Constant2/1 -> Switch/1
  Switch/1 -> Scope/1, MATLAB Function/1(t)  "t"
  Constant/1 -> MATLAB Function/2(f)
  MATLAB Function/2(y) -> y_traj/1, Sum7/2  "y_traj"
  Zero-Order Hold/1 -> Switch/2, Switch/3
  Constant1/1 -> MATLAB Function/3(scale)
  Constant3/1 -> MATLAB Function/4(sampling_time)
  MATLAB Function/1(x) -> x_traj/1, Sum3/2  "x_traj"
  MATLAB Function/3(psi) -> psi_traj/1  "psi_traj"
  Clock/1 -> Sum/1, Switch1/2
  Constant4/1 -> Switch1/3
  Switch1/1 -> Zero-Order Hold/1
  Constant5/1 -> Sum/2
  Sum/1 -> Switch1/1
  Constant6/1 -> MATLAB Function/5(total_time)
  Sum7/1 -> Abs1/1
  Abs/1 -> Sum9/1
  Abs1/1 -> Sum9/2
  [y] -> Sum7/1
  Sum9/1 -> Integrator/1
  Integrator/1 -> Scope1/1  "pos_err"
  [x] -> Sum3/1
  Sum3/1 -> Abs/1
  Constant7/1 -> MATLAB Function/6(start_time)

== system B5_simulation_paparazzi/Model Block Normal Filters/Simple INDI/Doublet Block ==
  Scope : Scope
  Step : Step  Time=start_time  After=doublet_mag  SampleTime=sampling_time
  Step1 : Step  Time=start_time + doublet_time/2  After=-doublet_mag*2  SampleTime=sampling_time
  Step2 : Step  Time=start_time + doublet_time  After=doublet_mag  SampleTime=sampling_time
  Sum : Sum  Inputs=|++
  Sum1 : Sum  Inputs=|++
  theta_cmd : Outport
  wires:
  Step/1 -> Sum/1
  Step1/1 -> Sum/2
  Sum/1 -> Sum1/1
  Sum1/1 -> theta_cmd/1, Scope/1
  Step2/1 -> Sum1/2

== system B5_simulation_paparazzi/Model Block Normal Filters/Simple INDI/ERROR CONTROLLER ATTITUDE ==
  p_ref : Inport
  q_ref : Inport  Port=2
  r_ref : Inport  Port=3
  phi_ref : Inport  Port=4
  theta_ref : Inport  Port=5
  psi_ref : Inport  Port=6
  Abs : Abs
  Add : Sum  Inputs=++++
  Add1 : Sum  Inputs=++++
  Add2 : Sum  Inputs=+++
  Cumulative Sum : dspmathops/Cumulative Sum  dim=Channels (running sum)  InputProcessing=Columns as channels (frame based)  reset_popup=None  roundingMode=Floor  overflowMode=off  outputDataTypeStr=Inherit: Same as accumulator  outputMin=[]  outputMax=[]  outputLastDataTypeStr=Inherit: Same as accumulator
  Discrete-Time Integrator : DiscreteIntegrator  SampleTime=-1  ICPrevOutput=DiscIntNeverNeededParam  ICPrevScaledInput=DiscIntNeverNeededParam
  Discrete-Time Integrator1 : DiscreteIntegrator  SampleTime=-1  ICPrevOutput=DiscIntNeverNeededParam  ICPrevScaledInput=DiscIntNeverNeededParam
  Discrete-Time Integrator2 : DiscreteIntegrator  SampleTime=-1  ICPrevOutput=DiscIntNeverNeededParam  ICPrevScaledInput=DiscIntNeverNeededParam
  Display : Display
  Display1 : Display
  Gain1 : Gain  Gain=K_ec_d
  Gain10 : Gain  Gain=K_ec_i
  Gain11 : Gain  Gain=K_ec_i
  Gain2 : Gain  Gain=K_ec
  Gain4 : Gain  Gain=K_ec_d
  Gain5 : Gain  Gain=K_ec
  Gain7 : Gain  Gain=K_ec_d
  Gain8 : Gain  Gain=K_ec
  Gain9 : Gain  Gain=K_ec_i
  MATLAB Function1 : MATLAB Function  TreatAsAtomicUnit=on
  Mean : dspstat3/Mean  run=off  InputProcessing=Columns as channels (frame based)  reset_popup=None  directionMode=Each column  dimension=1  roiEnable=off  roiType=Rectangles  roiPortion=Entire ROI  roiOutput=Individual statistics for each ROI  roiFlag=off  roundingMode=Floor  overflowMode=off  outputDataTypeStr=Inherit: Same as accumulator  outputMin=[]  outputMax=[]  outputLastDataTypeStr=Inherit: Same as accumulator
  Sum{1..2,4..5,7..8} (6 alike) : Sum  Inputs=|+-
  pd_ec : Outport
  qd_ec : Outport  Port=2
  rd_ec : Outport  Port=3
  wires:
  p_ref/1 -> Sum1/1
  Add/1 -> pd_ec/1
  [p] -> Sum1/2
  [phi] -> Sum2/2
  phi_ref/1 -> Sum2/1
  Sum1/1 -> Gain1/1  "p_err"
  Sum2/1 -> Discrete-Time Integrator1/1, Gain2/1  "phi_err"
  Gain1/1 -> Add/2
  Gain2/1 -> Add/3
  Sum4/1 -> Gain4/1  "q_err"
  Gain4/1 -> Add1/2
  Gain5/1 -> Add1/3
  theta_ref/1 -> Sum5/1
  [theta] -> Sum5/2
  [q] -> Sum4/2
  q_ref/1 -> Sum4/1
  Add1/1 -> qd_ec/1
  Sum7/1 -> Gain7/1  "r_err"
  Sum8/1 -> MATLAB Function1/1(pis_e)
  Gain7/1 -> Add2/2  "2"
  Gain8/1 -> Add2/3  "3"
  psi_ref/1 -> Sum8/1
  [psi] -> Sum8/2
  [r] -> Sum7/2
  r_ref/1 -> Sum7/1
  Add2/1 -> rd_ec/1
  Sum5/1 -> Abs/1, Discrete-Time Integrator/1, Gain5/1  "theta_err"
  MATLAB Function1/1(psie_w) -> Discrete-Time Integrator2/1, Gain8/1  "psi_err"
  Abs/1 -> Mean/1, Cumulative Sum/1  "theta_err_abs"
  Cumulative Sum/1 -> Display/1
  Mean/1 -> Display1/1
  Discrete-Time Integrator/1 -> Gain9/1
  Gain9/1 -> Add1/4
  Discrete-Time Integrator1/1 -> Gain10/1
  Gain10/1 -> Add/4
  Discrete-Time Integrator2/1 -> Gain11/1
  Gain11/1 -> Add2/1  "4"

== system B5_simulation_paparazzi/Model Block Normal Filters/Simple INDI/ERROR CONTROLLER VELOCITY ==
  Vx_ref : Inport
  Vy_ref : Inport  Port=2
  Vz_ref : Inport  Port=3
  X_ref : Inport  Port=4
  Y_ref : Inport  Port=5
  Z_ref : Inport  Port=6
  Gain : Gain  Gain=K_ec_u
  Gain1 : Gain  Gain=K_ec_d_u
  Gain2 : Gain  Gain=K_ec_v
  Gain3 : Gain  Gain=K_ec_d_v
  Gain4 : Gain  Gain=K_ec_v
  Gain5 : Gain  Gain=K_ec_d_v
  Sum{,3,5..8} (6 alike) : Sum  Inputs=|+-
  Sum1 : Sum  Inputs=|++
  Sum2 : Sum  Inputs=|++
  Sum4 : Sum  Inputs=|++
  Ax_ec : Outport
  Ay_ec : Outport  Port=2
  Az_ec : Outport  Port=3
  wires:
  [Vz] -> Sum6/2
  Sum1/1 -> Ax_ec/1
  Sum2/1 -> Ay_ec/1
  Vy_ref/1 -> Sum3/1
  Vx_ref/1 -> Sum/1
  [Vy] -> Sum3/2
  Vz_ref/1 -> Sum6/1
  Sum/1 -> Gain1/1  "Vx_error"
  Sum4/1 -> Az_ec/1
  [Vx] -> Sum/2
  [x] -> Sum5/2
  X_ref/1 -> Sum5/1
  Sum5/1 -> Gain/1
  Gain1/1 -> Sum1/1
  Gain/1 -> Sum1/2
  Gain3/1 -> Sum2/1
  Sum3/1 -> Gain3/1  "Vy_error"
  Gain5/1 -> Sum4/1
  Sum6/1 -> Gain5/1  "Vz_error"
  Y_ref/1 -> Sum7/1
  [y] -> Sum7/2
  Sum7/1 -> Gain2/1
  Z_ref/1 -> Sum8/1
  [z] -> Sum8/2
  Sum8/1 -> Gain4/1
  Gain4/1 -> Sum4/2
  Gain2/1 -> Sum2/2

== system B5_simulation_paparazzi/Model Block Normal Filters/Simple INDI/INTERNAL REFERENCE MODEL ATTITUDE ==
  phi_cmd : Inport
  theta_cmd : Inport  Port=2
  psi_cmd : Inport  Port=3
  Discrete-Time Integrator{,1..5} (6 alike) : DiscreteIntegrator  SampleTime=sampling_time  ICPrevOutput=DiscIntNeverNeededParam  ICPrevScaledInput=DiscIntNeverNeededParam
  Gain1 : Gain  Gain=K
  Gain3 : Gain  Gain=K
  Gain4 : Gain  Gain=K_d
  Gain5 : Gain  Gain=K_d
  Gain6 : Gain  Gain=K_d
  Gain7 : Gain  Gain=K
  MATLAB Function1 : MATLAB Function  TreatAsAtomicUnit=on
  Mux : Mux  Inputs=6
  Scope : Scope  NumInputPorts=2
  Sum{1,11,16,20..22} (6 alike) : Sum  Inputs=|+-
  To Workspace : ToWorkspace  VariableName=indi  SaveFormat=Timeseries  SampleTime=-1
  body rates to euler rates : Subsystem
  euler rates to body rates : Subsystem
  pd_ref : Outport
  qd_ref : Outport  Port=2
  rd_ref : Outport  Port=3
  p_ref : Outport  Port=4
  q_ref : Outport  Port=5
  r_ref : Outport  Port=6
  phi_ref : Outport  Port=7
  theta_ref : Outport  Port=8
  psi_ref : Outport  Port=9
  tag scope: p_ref=global, phi_ref=global, psi_ref=global, q_ref=global, r_ref=global, theta_ref=global
  wires:
  Discrete-Time Integrator1/1 -> [theta_ref], Mux/3, theta_ref/1, Sum11/2  "theta_ref"
  Gain6/1 -> Discrete-Time Integrator5/1, rd_ref/1  "rd_ref"
  Discrete-Time Integrator3/1 -> Sum21/2, [p_ref], p_ref/1, body rates to euler rates/1(p)  "p_ref"
  Discrete-Time Integrator5/1 -> [r_ref], r_ref/1, body rates to euler rates/3(r), Sum22/2  "r_ref"
  Discrete-Time Integrator4/1 -> Scope/1, body rates to euler rates/2(q), [q_ref], Mux/2, q_ref/1, Sum16/2  "q_ref"
  Gain5/1 -> Discrete-Time Integrator4/1, Mux/1, qd_ref/1  "qd_ref"
  Sum21/1 -> Gain4/1
  Sum11/1 -> Gain1/1
  Sum22/1 -> Gain6/1
  Sum16/1 -> Gain5/1
  Discrete-Time Integrator2/1 -> [phi_ref], phi_ref/1, Sum20/2  "phi_ref"
  Sum20/1 -> Gain7/1
  Gain4/1 -> Discrete-Time Integrator3/1, pd_ref/1  "pd_ref"
  phi_cmd/1 -> Sum20/1  "phi_cmd"
  theta_cmd/1 -> Sum11/1  "theta_cmd"
  psi_cmd/1 -> Sum1/1  "psi_cmd"
  Discrete-Time Integrator/1 -> [psi_ref], psi_ref/1, Sum1/2  "psi_ref"
  Sum1/1 -> MATLAB Function1/1(pis_e)  "err"
  Gain7/1 -> euler rates to body rates/1(phi_dot)
  euler rates to body rates/1(p) -> Sum21/1
  Gain1/1 -> euler rates to body rates/2(theta_dot)
  euler rates to body rates/2(q) -> Sum16/1
  Gain3/1 -> euler rates to body rates/3(psi_dot)
  euler rates to body rates/3(r) -> Sum22/1
  body rates to euler rates/3(psi_dot) -> Discrete-Time Integrator/1
  body rates to euler rates/2(theta_dot) -> Scope/2, Discrete-Time Integrator1/1
  body rates to euler rates/1(phi_dot) -> Discrete-Time Integrator2/1
  MATLAB Function1/1(psie_w) -> Gain3/1  "wrapped_Err"
  Mux/1 -> To Workspace/1
  [qd_f] -> Mux/4
  [theta] -> Mux/6
  [q] -> Mux/5

== system B5_simulation_paparazzi/Model Block Normal Filters/Simple INDI/INTERNAL REFERENCE MODEL VELOCITY ==
  Vx_cmd : Inport
  Vy_cmd : Inport  Port=2
  Vz_cmd : Inport  Port=3
  Discrete-Time Integrator{,1..5} (6 alike) : DiscreteIntegrator  SampleTime=-1  ICPrevOutput=DiscIntNeverNeededParam  ICPrevScaledInput=DiscIntNeverNeededParam
  Gain1 : Gain  Gain=K_w_d
  Gain2 : Gain  Gain=K_v_d
  Gain3 : Gain  Gain=K_w
  Gain4 : Gain  Gain=K_v
  Gain5 : Gain  Gain=K_u
  Gain9 : Gain  Gain=K_u_d
  Sum{1..4,11,20} (6 alike) : Sum  Inputs=|+-
  Ax_ref : Outport
  Ay_ref : Outport  Port=2
  Az_ref : Outport  Port=3
  Vx_ref : Outport  Port=4
  Vy_ref : Outport  Port=5
  Vz_ref : Outport  Port=6
  X_ref : Outport  Port=7
  Y_ref : Outport  Port=8
  Z_ref : Outport  Port=9
  tag scope: Ax_ref=global, Ay_ref=global, Az_ref=global, Vx_ref=global, Vy_ref=global, Vz_ref=global
  wires:
  Discrete-Time Integrator1/1 -> Sum3/2, Discrete-Time Integrator4/1, [Vy_ref], Vz_ref/1
  Gain1/1 -> Discrete-Time Integrator1/1, [Az_ref], Az_ref/1
  Gain9/1 -> Discrete-Time Integrator/1, [Ax_ref], Ax_ref/1
  Vy_cmd/1 -> Sum1/1
  Discrete-Time Integrator/1 -> Sum4/2, Discrete-Time Integrator3/1, [Vx_ref], Vx_ref/1
  Vx_cmd/1 -> Sum20/1
  Vz_cmd/1 -> Sum11/1
  Discrete-Time Integrator2/1 -> Sum2/2, Discrete-Time Integrator5/1, [Vz_ref], Vy_ref/1
  Gain2/1 -> Discrete-Time Integrator2/1, [Ay_ref], Ay_ref/1
  Sum20/1 -> Gain5/1
  Sum11/1 -> Gain3/1
  Sum1/1 -> Gain4/1
  Gain4/1 -> Sum2/1
  Gain3/1 -> Sum3/1
  Gain5/1 -> Sum4/1
  Sum3/1 -> Gain1/1
  Sum2/1 -> Gain2/1
  Sum4/1 -> Gain9/1
  Discrete-Time Integrator3/1 -> X_ref/1, Sum20/2
  Discrete-Time Integrator4/1 -> Sum11/2, Z_ref/1
  Discrete-Time Integrator5/1 -> Sum1/2, Y_ref/1

== system B5_simulation_paparazzi/Model Block Complementary Filters/Continuous Actuator Dynamics/Noise RPM/Switch Case Action Subsystem ==
  Action Port : ActionPort  ActionPortLabel=case [ 1 ]:
  RPM Noise : simulink/Sources/Band-Limited White Noise  Cov=[NOISE_RPM]  Ts=sampling_time  seed=[23341]
  Out1 : Outport
  wires:
  RPM Noise/1 -> Out1/1

== system B5_simulation_paparazzi/Model Block Complementary Filters/Continuous Actuator Dynamics/Noise RPM/Switch Case Action Subsystem1 ==
  Action Port : ActionPort  ActionPortLabel=default:
  Constant : Constant  Value=0  SampleTime=sampling_time
  Out1 : Outport
  wires:
  Constant/1 -> Out1/1

== system B5_simulation_paparazzi/Model Block Complementary Filters/Extended INDI/INTERNAL REFERENCE MODEL ATTITUDE/body rates to euler rates ==
  p : Inport
  q : Inport  Port=2
  r : Inport  Port=3
  Demux : Demux  Outputs=3
  Matrix Multiply : Product  Multiplication=Matrix(*)
  Mux : Mux  Inputs=3
  phi_dot : Outport
  theta_dot : Outport  Port=2
  psi_dot : Outport  Port=3
  wires:
  p/1 -> Mux/1
  q/1 -> Mux/2
  r/1 -> Mux/3
  [T_discr] -> Matrix Multiply/1
  Mux/1 -> Matrix Multiply/2
  Matrix Multiply/1 -> Demux/1
  Demux/3 -> psi_dot/1
  Demux/2 -> theta_dot/1
  Demux/1 -> phi_dot/1

== system B5_simulation_paparazzi/Model Block Complementary Filters/Extended INDI/INTERNAL REFERENCE MODEL ATTITUDE/euler rates to body rates ==
  phi_dot : Inport
  theta_dot : Inport  Port=2
  psi_dot : Inport  Port=3
  Demux : Demux  Outputs=3
  Matrix Multiply : Product  Multiplication=Matrix(*)
  Mux : Mux  Inputs=3
  p : Outport
  q : Outport  Port=2
  r : Outport  Port=3
  wires:
  phi_dot/1 -> Mux/1
  theta_dot/1 -> Mux/2
  psi_dot/1 -> Mux/3
  [R_discr] -> Matrix Multiply/1
  Mux/1 -> Matrix Multiply/2
  Matrix Multiply/1 -> Demux/1
  Demux/3 -> r/1
  Demux/2 -> q/1
  Demux/1 -> p/1

== system B5_simulation_paparazzi/Model Block Complementary Filters/Extended INDI/Subsystem/body rates to euler rates ==
  p : Inport
  q : Inport  Port=2
  r : Inport  Port=3
  Demux : Demux  Outputs=3
  Matrix Multiply : Product  Multiplication=Matrix(*)
  Mux : Mux  Inputs=3
  phi_dot : Outport
  theta_dot : Outport  Port=2
  psi_dot : Outport  Port=3
  wires:
  p/1 -> Mux/1
  q/1 -> Mux/2
  r/1 -> Mux/3
  [T_discr] -> Matrix Multiply/1
  Mux/1 -> Matrix Multiply/2
  Matrix Multiply/1 -> Demux/1
  Demux/3 -> psi_dot/1
  Demux/2 -> theta_dot/1
  Demux/1 -> phi_dot/1

== system B5_simulation_paparazzi/Model Block Complementary Filters/Plant and State Estimation/Angular Velocity Model/Drag Plate Aerodynamics ==
  Constant : Constant  Value=0  SampleTime=sampling_time
  Constant1 : Constant  Value=w_plate
  Constant4 : Constant  Value=h_plate
  Constant6 : Constant  Value=l_plate
  Mux : Mux  Inputs=3
  Scope1 : Scope  NumInputPorts=3
  Scope2 : Scope  NumInputPorts=2
  Scope3 : Scope  NumInputPorts=3
  Scope4 : Scope
  Scope5 : Scope  NumInputPorts=3
  drag plate My1 : MATLAB Function  TreatAsAtomicUnit=on
  aero_moment : Outport
  wires:
  Constant4/1 -> drag plate My1/2(h_plate)
  Constant6/1 -> drag plate My1/3(l_plate)
  [theta_cont] -> drag plate My1/4("theta ")
  Constant1/1 -> drag plate My1/1(w_plate)
  [Vy_cont] -> drag plate My1/6("Vy ")
  [Vx_cont] -> drag plate My1/5("Vx ")
  drag plate My1/6(gamma) -> Scope1/1  "gamma"
  [Vz_cont] -> drag plate My1/7("Vz ")
  drag plate My1/7(theta) -> Scope1/2  "theta_deg"
  drag plate My1/8(alpha) -> Scope1/3  "alpha"
  drag plate My1/1(Cd) -> Scope2/1  "Cd"
  drag plate My1/2(Cl) -> Scope2/2  "Cl"
  drag plate My1/9(D_plate) -> Scope3/1  "D_plate"
  drag plate My1/10(L_plate) -> Scope3/2  "L_plate"
  [u_cont] -> drag plate My1/8(u)
  drag plate My1/12(My_dp) -> Mux/2, Scope4/1  "My_dp"
  drag plate My1/3(Vx) -> Scope5/1  "Vx"
  drag plate My1/4(Vy) -> Scope5/2  "Vy"
  drag plate My1/5(Vz) -> Scope5/3  "Vz"
  Constant/1 -> Mux/1, Mux/3
  Mux/1 -> aero_moment/1
  drag plate My1/11(R_plate) -> Scope3/3  "R_plate"

== system B5_simulation_paparazzi/Model Block Complementary Filters/Plant and State Estimation/Complementary Filter/Butterworth Lowpass 2nd Order1 ==
  In : Inport
  Constant : Constant  Value=FILTER  SampleTime=sampling_time
  Merge : Merge
  Switch Case : SwitchCase
  Switch Case Action Subsystem : Subsystem  TreatAsAtomicUnit=on
  Switch Case Action Subsystem1 : Subsystem  TreatAsAtomicUnit=on
  Out : Outport
  wires:
  Merge/1 -> Out/1
  Switch Case Action Subsystem/1(Out1) -> Merge/1
  Constant/1 -> Switch Case/1
  Switch Case Action Subsystem1/1(Out1) -> Merge/2
  Switch Case/2 -> Switch Case Action Subsystem1/Action
  In/1 -> Switch Case Action Subsystem/1(In1), Switch Case Action Subsystem1/1(In1)
  Switch Case/1 -> Switch Case Action Subsystem/Action

== system B5_simulation_paparazzi/Model Block Complementary Filters/Plant and State Estimation/Complementary Filter/Butterworth Lowpass 2nd Order2 ==
  In : Inport
  Constant : Constant  Value=FILTER  SampleTime=sampling_time
  Merge : Merge
  Switch Case : SwitchCase
  Switch Case Action Subsystem : Subsystem  TreatAsAtomicUnit=on
  Switch Case Action Subsystem1 : Subsystem  TreatAsAtomicUnit=on
  Out : Outport
  wires:
  Merge/1 -> Out/1
  Switch Case Action Subsystem/1(Out1) -> Merge/1
  Constant/1 -> Switch Case/1
  Switch Case Action Subsystem1/1(Out1) -> Merge/2
  Switch Case/2 -> Switch Case Action Subsystem1/Action
  In/1 -> Switch Case Action Subsystem/1(In1), Switch Case Action Subsystem1/1(In1)
  Switch Case/1 -> Switch Case Action Subsystem/Action
